simulink model "problem_controller"  (R2020b)
settings: Solver=FixedStepAuto  StartTime=0.0  StopTime=10.0  RelTol=1e-3
undefined symbols (not defined in the file): Kd, Ki, Kp, N
settings Model: DataDictionary=data_dic.sldd  Creator=Gopinath Murugan  LastModifiedBy=Gopinath Murugan

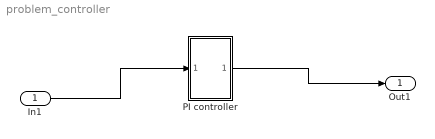
== system problem_controller ==
  In1 : Inport
  PI controller : Subsystem
  Out1 : Outport
  wires:
  In1/1 -> PI controller/1(In1)
  PI controller/1(Out1) -> Out1/1

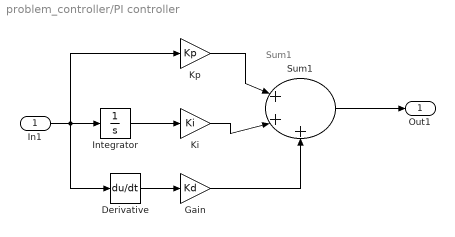
== system problem_controller/PI controller ==
  note: Sum1
  In1 : Inport
  Derivative : Derivative  CoefficientInTFapproximation=1/N
  Gain : Gain  Gain=Kd
  Integrator : Integrator
  Ki : Gain  Gain=Ki
  Kp : Gain  Gain=Kp
  Sum1 : Sum  Inputs=|+++
  Out1 : Outport
  wires:
  Kp/1 -> Sum1/1
  Integrator/1 -> Ki/1
  In1/1 -> Derivative/1, Kp/1, Integrator/1
  Ki/1 -> Sum1/2
  Sum1/1 -> Out1/1
  Derivative/1 -> Gain/1
  Gain/1 -> Sum1/3
